simulink model "model_skidpad"  (R2023b)
settings: Solver=FixedStepAuto  StartTime=0.0  StopTime=200  FixedStep=0.005  RelTol=1e-3
values from neighbouring files (symbols this model uses):
  A_sim = [(-CF-CR)/(m*Vv),(-CF*a+CR*b-m*Vv^2)/(m*Vv^2) ... (first row only)    [main.m]    (also in main_skidpad.m)
  B_sim = [CF/(m*Vv) -CR/(m*Vv) ... (first row only)    [main.m]    (also in main_skidpad.m)
  C = eye(4)    [main.m]    (also in main_skidpad.m; single_track_model_analysis.m = [1,0)
  C_sim = [1,0 ... (first row only)    [main.m]    (also in main_skidpad.m)
  D_sim = [0 0 ... (first row only)    [main.m]    (also in main_skidpad.m)
  delta_max = 25    [load_params.m]    (also in main.m; main_skidpad.m)
  Kff = m*Vxb^2/l*(lr/Cf-lf/Cr+lf/Cr*K(3))+l-lr*K(3)    [main.m]    (also in main_skidpad.m = zeros(200,1))
libraries: simulink_extras x6, simulink x1
settings Model: Creator=edoardocavallotti  LastModifiedBy=edoardocavallotti

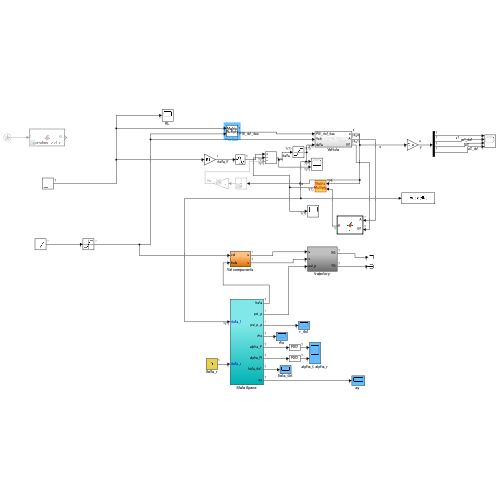
[thumbnail: Simulink's stored preview of the top-level diagram]
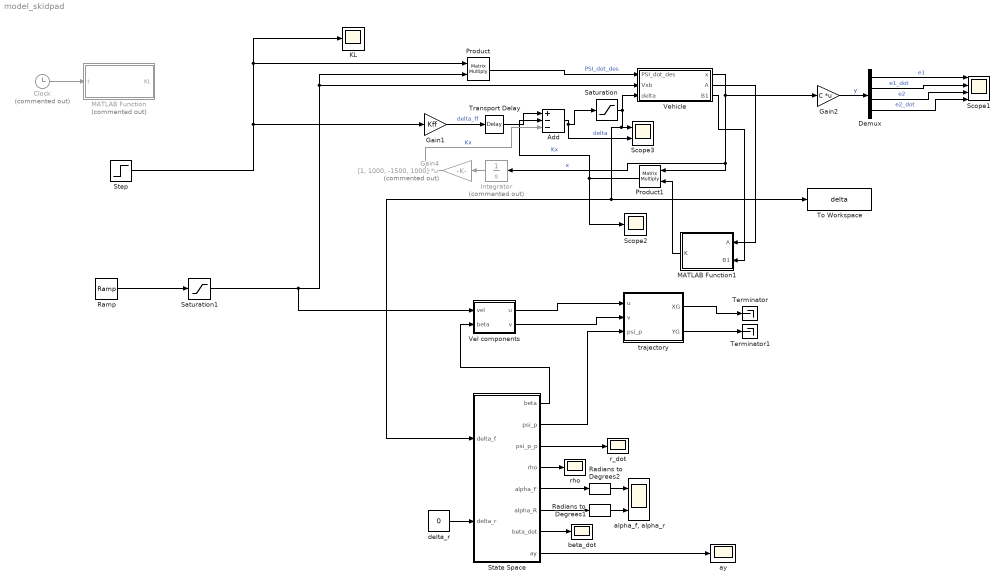
== system model_skidpad ==
  Add : Sum  Inputs=+--
  Clock : Clock  Commented=on
  Demux : Demux
  Gain1 : Gain  Gain=Kff
  Gain2 : Gain  Gain=C  Multiplication=Matrix(K*u)
  Gain4 : Gain  Commented=on  Gain=[1, 1000, -1500, 1000]  Multiplication=Matrix(K*u)
  Integrator : Integrator  Commented=on  InitialCondition=zeros(4,1)
  KL : Scope
  MATLAB Function : MATLAB Function  Commented=on  TreatAsAtomicUnit=on
  MATLAB Function1 : MATLAB Function  TreatAsAtomicUnit=on
  Product : Product  Multiplication=Matrix(*)
  Product1 : Product  Multiplication=Matrix(*)
  Radians to Degrees1 : simulink_extras/Transformations/Radians to Degrees
  Radians to Degrees2 : simulink_extras/Transformations/Radians to Degrees
  Ramp : simulink/Sources/Ramp  slope=1  start=0  InitialOutput=10
  Saturation : Saturate  UpperLimit=delta_max  LowerLimit=-delta_max
  Saturation1 : Saturate  UpperLimit=35  LowerLimit=-inf
  Scope1 : Scope  NumInputPorts=4
  Scope2 : Scope
  Scope3 : Scope  NumInputPorts=2
  State Space : Subsystem
  Step : Step  Time=0.5  After=0.02  SampleTime=0
  Terminator : Terminator
  Terminator1 : Terminator
  To Workspace : ToWorkspace  VariableName=delta  SaveFormat=Timeseries  SampleTime=-1
  Transport Delay : TransportDelay  DelayTime=0.01
  Vehicle : Subsystem
  Vel components : Subsystem
  "alpha_f, alpha_r" : Scope  NumInputPorts=2
  "ay " : Scope
  beta_dot : Scope
  delta_r : Constant  Value=0
  r_dot : Scope
  rho : Scope
  trajectory : Subsystem
  wires:
  Add/1 -> Scope3/2, Saturation/1  "delta"
  Vehicle/1(x) -> Product1/1, Integrator/1, Gain2/1  "x"
  Product1/1 -> Scope2/1, Add/2  "Kx"
  Product/1 -> Vehicle/1(PSI_dot_des)  "PSI_dot_des"
  Gain1/1 -> Transport Delay/1  "delta_ff"
  Gain2/1 -> Demux/1  "y"
  Demux/1 -> Scope1/1  "e1"
  Demux/2 -> Scope1/2  "e1_dot"
  Demux/3 -> Scope1/3  "e2"
  Demux/4 -> Scope1/4  "e2_dot"
  Radians to Degrees1/1 -> "alpha_f, alpha_r"/2
  State Space/2(psi_p) -> trajectory/3(psi_p)
  delta_r/1 -> State Space/2(delta_r)
  State Space/7("beta_dot ") -> beta_dot/1
  Saturation1/1 -> Vehicle/2(Vxb), Product/2, Vel components/1(vel)
  State Space/5(alpha_F) -> Radians to Degrees2/1
  State Space/1(beta) -> Vel components/2(beta)
  State Space/8(ay) -> "ay "/1
  Vel components/1(u) -> trajectory/1(u)
  State Space/6(alpha_R) -> Radians to Degrees1/1
  State Space/3(psi_p_p) -> r_dot/1
  trajectory/1(XG) -> Terminator/1
  State Space/4(rho) -> rho/1
  trajectory/2(YG) -> Terminator1/1
  Vel components/2(v) -> trajectory/2(v)
  Radians to Degrees2/1 -> "alpha_f, alpha_r"/1
  Transport Delay/1 -> Add/1
  Saturation/1 -> To Workspace/1, State Space/1(delta_f), Scope3/1, Vehicle/3(delta)
  Integrator/1 -> Gain4/1
  Gain4/1 -> Add/3  "Kx"
  Clock/1 -> MATLAB Function/1(t)
  Step/1 -> Product/1, KL/1, Gain1/1
  Ramp/1 -> Saturation1/1
  Vehicle/2(A) -> MATLAB Function1/1(A)
  Vehicle/3(B1) -> MATLAB Function1/2(B1)
  MATLAB Function1/1(K) -> Product1/2

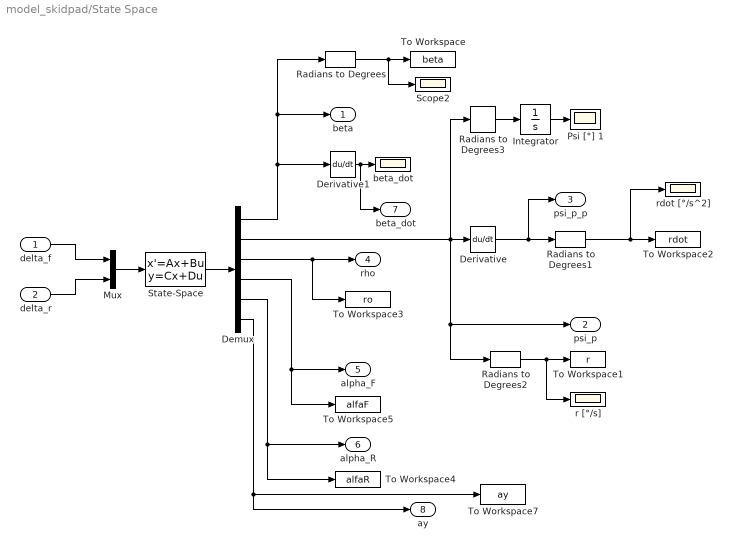
== system model_skidpad/State Space ==
  delta_f : Inport
  delta_r : Inport  Port=2
  Demux : Demux  Outputs=6
  Derivative : Derivative
  Derivative1 : Derivative
  Integrator : Integrator
  Mux : Mux  Inputs=2
  Psi [°] 1 : Scope
  Radians to Degrees{,1..3} (4 alike) : simulink_extras/Transformations/Radians to Degrees
  Scope2 : Scope
  State-Space : StateSpace  A=A_sim  B=B_sim  C=C_sim  D=D_sim  InitialCondition=0
  To Workspace : ToWorkspace  VariableName=beta  SaveFormat=Timeseries  SampleTime=-1
  To Workspace1 : ToWorkspace  VariableName=r  SaveFormat=Timeseries  SampleTime=-1
  To Workspace2 : ToWorkspace  VariableName=rdot  SaveFormat=Timeseries  SampleTime=-1
  To Workspace3 : ToWorkspace  VariableName=ro  SaveFormat=Timeseries  SampleTime=-1
  To Workspace4 : ToWorkspace  VariableName=alfaR  SaveFormat=Timeseries  SampleTime=-1
  To Workspace5 : ToWorkspace  VariableName=alfaF  SaveFormat=Timeseries  SampleTime=-1
  To Workspace7 : ToWorkspace  VariableName=ay  SaveFormat=Timeseries  SampleTime=-1
      settings: Save2DSignal=2-D array (concatenate along first dimension)
  beta_dot : Scope
  r [°/s] : Scope
  rdot [°/s^2] : Scope
  beta : Outport  VectorParamsAs1DForOutWhenUnconnected=off
  psi_p : Outport  Port=2  VectorParamsAs1DForOutWhenUnconnected=off
  psi_p_p : Outport  Port=3  VectorParamsAs1DForOutWhenUnconnected=off
  rho : Outport  Port=4  VectorParamsAs1DForOutWhenUnconnected=off
  alpha_F : Outport  Port=5  VectorParamsAs1DForOutWhenUnconnected=off
  alpha_R : Outport  Port=6  VectorParamsAs1DForOutWhenUnconnected=off
  "beta_dot " : Outport  Port=7  VectorParamsAs1DForOutWhenUnconnected=off
  ay : Outport  Port=8  VectorParamsAs1DForOutWhenUnconnected=off
  wires:
  Demux/2 -> psi_p/1, Radians to Degrees2/1, Radians to Degrees3/1, Derivative/1
  Demux/1 -> Derivative1/1, beta/1, Radians to Degrees/1
  Derivative/1 -> Radians to Degrees1/1, psi_p_p/1
  Radians to Degrees/1 -> Scope2/1, To Workspace/1
  Radians to Degrees1/1 -> rdot [°/s^2]/1, To Workspace2/1
  Radians to Degrees2/1 -> r [°/s]/1, To Workspace1/1
  Demux/3 -> To Workspace3/1, rho/1
  Demux/4 -> alpha_F/1, To Workspace5/1
  Demux/5 -> To Workspace4/1, alpha_R/1
  Radians to Degrees3/1 -> Integrator/1
  Integrator/1 -> Psi [°] 1/1
  Derivative1/1 -> "beta_dot "/1, beta_dot/1
  delta_f/1 -> Mux/1
  delta_r/1 -> Mux/2
  Demux/6 -> ay/1, To Workspace7/1
  Mux/1 -> State-Space/1
  State-Space/1 -> Demux/1

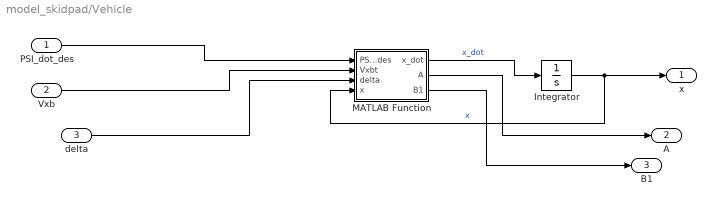
== system model_skidpad/Vehicle ==
  PSI_dot_des : Inport
  Vxb : Inport  Port=2
  delta : Inport  Port=3
  Integrator : Integrator  InitialCondition=zeros(4,1)
  MATLAB Function : MATLAB Function  TreatAsAtomicUnit=on
  x : Outport
  A : Outport  Port=2
  B1 : Outport  Port=3
  wires:
  Integrator/1 -> MATLAB Function/4(x), x/1  "x"
  MATLAB Function/1(x_dot) -> Integrator/1  "x_dot"
  PSI_dot_des/1 -> MATLAB Function/1(PSI_dot_des)
  Vxb/1 -> MATLAB Function/2(Vxbt)
  delta/1 -> MATLAB Function/3(delta)
  MATLAB Function/2(A) -> A/1
  MATLAB Function/3(B1) -> B1/1

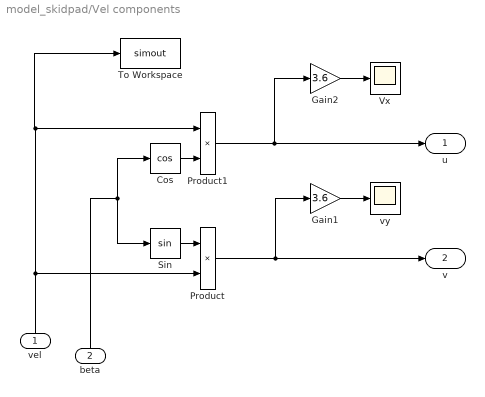
== system model_skidpad/Vel components ==
  vel : Inport
  beta : Inport  Port=2
  Cos : Trigonometry  Operator=cos
  Gain1 : Gain  Gain=3.6
  Gain2 : Gain  Gain=3.6
  Product : Product
  Product1 : Product
  Sin : Trigonometry
  To Workspace : ToWorkspace  VariableName=simout  SaveFormat=Timeseries  SampleTime=-1
  Vx : Scope
  vy : Scope
  u : Outport  VectorParamsAs1DForOutWhenUnconnected=off
  v : Outport  Port=2  VectorParamsAs1DForOutWhenUnconnected=off
  wires:
  Product/1 -> Gain1/1, v/1
  vel/1 -> Product/2, Product1/1, To Workspace/1
  Gain1/1 -> vy/1
  Gain2/1 -> Vx/1
  Cos/1 -> Product1/2
  Product1/1 -> Gain2/1, u/1
  beta/1 -> Sin/1, Cos/1
  Sin/1 -> Product/1

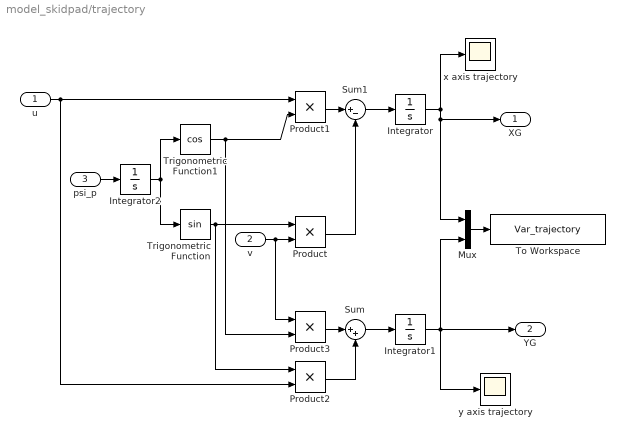
== system model_skidpad/trajectory ==
  u : Inport
  v : Inport  Port=2
  psi_p : Inport  Port=3
  Integrator : Integrator
  Integrator1 : Integrator  InitialCondition=1000
  Integrator2 : Integrator
  Mux : Mux  Inputs=2
  Product{,1..3} (4 alike) : Product  InputSameDT=on  SaturateOnIntegerOverflow=on  OutDataTypeStr=Inherit: Same as first input
  Sum : Sum  Inputs=|++  InputSameDT=on  SaturateOnIntegerOverflow=on  OutDataTypeStr=Inherit: Same as first input
  Sum1 : Sum  Inputs=|+-  InputSameDT=on  SaturateOnIntegerOverflow=on  OutDataTypeStr=Inherit: Same as first input
  To Workspace : ToWorkspace  VariableName=Var_trajectory  SampleTime=-1
      settings: Save2DSignal=2-D array (concatenate along first dimension)
      settings: InitFcn=|
      | ParentName = get_param(gcb,'Parent');
      | cont = max(find(ParentName=='/'));
      | set_param(gcb,'VariableName',strcat('Var_',ParentName(cont+1:length(ParentName))));
      | clear ParentName cont
  Trigonometric Function : Trigonometry
  Trigonometric Function1 : Trigonometry  Operator=cos
  x axis trajectory : Scope
  y axis trajectory : Scope
  XG : Outport  VectorParamsAs1DForOutWhenUnconnected=off
  YG : Outport  Port=2  VectorParamsAs1DForOutWhenUnconnected=off
  wires:
  psi_p/1 -> Integrator2/1
  Product1/1 -> Sum1/1
  Product/1 -> Sum1/2
  Sum1/1 -> Integrator/1
  Trigonometric Function/1 -> Product/1, Product2/1
  u/1 -> Product2/2, Product1/1
  v/1 -> Product/2, Product3/1
  Trigonometric Function1/1 -> Product1/2, Product3/2
  Product3/1 -> Sum/1
  Product2/1 -> Sum/2
  Sum/1 -> Integrator1/1
  Integrator/1 -> XG/1, Mux/1, x axis trajectory/1
  Integrator1/1 -> YG/1, y axis trajectory/1, Mux/2
  Mux/1 -> To Workspace/1
  Integrator2/1 -> Trigonometric Function/1, Trigonometric Function1/1

== matlab function model_skidpad/Vehicle/MATLAB Function ==
  data: PSI_dot_des input; x_dot output; Vxbt input; delta input; x input; A output; B1 output
function [x_dot, A, B1] = fcn(PSI_dot_des, Vxbt, delta, x)

m = 1575;
Jpsi = 2875;
Jz = Jpsi;
lf = 1.3;
a = lf;
lr = 1.5;
b = lr;
Cf = 2*60e3;
%Cr = 2*57e3;
%Cr = 57e3; %over
Cr = Cf*a/b;

A = [0 1 0 0 
    0 -(Cf+Cr)/(m*Vxbt) (Cf+Cr)/m (Cr*lr-Cf*lf)/(m*Vxbt)
    0 0 0 1
    0 (Cr*lr-Cf*lf)/(Jpsi*Vxbt) (-Cr*lr+Cf*lf)/Jpsi -(Cr*lr^2+Cf*lf^2)/(Jpsi*Vxbt)];

B1 = [0
    Cf/m
    0
    Cf*lf/Jpsi];

B2 = [0
    (Cr*lr-Cf*lf)/(m*Vxbt)-Vxbt
    0
    -(Cr*lr^2+Cf*lf^2)/(Jpsi*Vxbt)];



x_dot = A*x + B1.*PSI_dot_des + B2.*delta;

== matlab function model_skidpad/MATLAB Function ==
  data: t input; KL output
function KL = curvature_profile(t)

KL = 0;

if t<=10 || t >=150 
    KL = 0;
elseif t>10 && t<=20
    KL = 2e-3*(t-10);
elseif t>20 && t<=140
    KL = 2e-2;
elseif t>140 && t<150
    KL = 2e-2-(t-140)*2e-3;

end

== matlab function model_skidpad/MATLAB Function1 ==
  data: A input; K output; B1 input
function K = fcn(A, B1)

K = acker(A, B1, [-1, -1, -1, -1]');

end
